simulink model "pll_hogge_lock"  (Simulink 6.6)
settings: Solver=ode23tb  StartTime=0.0  StopTime=200.0e-9  MaxStep=1.0e-12  RelTol=1e-4
values from neighbouring files (symbols this model uses):
  C1 = 2.2e-9    (= 2.2e-09)    [plot_bode_open_and_closed_2.m]    (also in plot_bode_open_and_closed_hogge.m)
  C2 = 1.0e-9    (= 1e-09)    [plot_bode_open_and_closed_1.m]    (also in plot_bode_open_and_closed_2.m = 3.3e-08; plot_bode_open_and_closed_hogge.m = 3.3e-08)
  R1 = 10000    [plot_bode_open_and_closed_1.m]
libraries: powerlib x8, simulink_extras x3, commsynccomp2 x1, simulink x1, dspswit3 x1
settings Model: Creator=Administrator  LastModifiedBy=Administrator

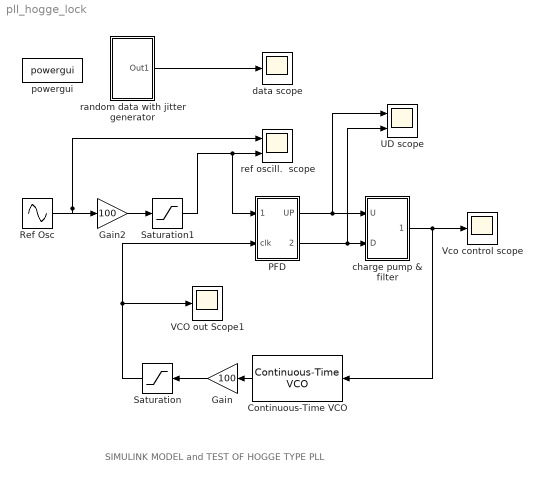
== system pll_hogge_lock ==
  note: SIMULINK MODEL and TEST OF HOGGE TYPE PLL
  " charge pump & filter" : Subsystem
  Continuous-Time VCO : commsynccomp2/Continuous-Time VCO  Orientation=left  SystemSampleTime=-1  Ac=1  Fc=1.999e9  Kc=500e6  Ph=-pi/2
  Gain : Gain  Orientation=left  Gain=100  RndMeth=Nearest
  Gain2 : Gain  Gain=100  RndMeth=Nearest
  PFD : Subsystem
  Ref Osc : Sin  Frequency=2*pi*1e9  Phase=3*pi/2  SampleTime=0
      settings: AttributesFormatString=%<Frequency> (rad/s)
  Saturation : Saturate  Orientation=left  UpperLimit=1  LowerLimit=0
  Saturation1 : Saturate  UpperLimit=1  LowerLimit=0
  UD scope : Scope  NumInputPorts=2
      settings: TimeRange=4.693877551020409e-008  YMin=-0.5~-0.5  YMax=1.5~1.5  SaveName=ScopeData5
  VCO out Scope1 : Scope
      settings: TimeRange=6.548881036513545e-009  YMin=-0.5  YMax=1.5  SaveName=ScopeData2  SampleTime=1e-8
  Vco control scope : Scope
      settings: TimeRange=2.564935064935065e-008  YMin=-0.8  YMax=1.2
  data scope : Scope
      settings: YMin=-0.5  YMax=1.5
  powergui : powerlib/powergui  SystemSampleTime=-1  SimulationMode=Continuous  SampleTime=50e-6  echomessages=off  RestoreLinks=warning  x0status=blocks  Frange=[0:2:500]  Ylog=off  Xlog=on  ShowGrid=off  save=off  variable=ZData  ZoomFFT=on  StartTime=0.0  cycles=1  DisplayStyle=1  fundamental=60  FreqAxis=off  MaxFrequency=1000  frequencyindice=0  frequencyindicesteady=1  RmsSteady=1  display=off  Ts=0  frequency=60  methode=off  HookPort=off  Interpol=off
  random data with jitter generator : Subsystem
  ref oscill.  scope : Scope  NumInputPorts=2
      settings: TimeRange=1.752837326607819e-008  YMin=-1.5~-0.5  YMax=1.5~1.5  SaveName=ScopeData3
  wires:
  random data with jitter generator/1(Out1) -> data scope/1
  Continuous-Time VCO/1 -> Gain/1
  PFD/1(UP) -> " charge pump & filter"/1(U), UD scope/1
  PFD/2(DN) -> " charge pump & filter"/2(D), UD scope/2
  " charge pump & filter"/1(contrl) -> Vco control scope/1, Continuous-Time VCO/1
  Ref Osc/1 -> ref oscill.  scope/1, Gain2/1
  Saturation/1 -> VCO out Scope1/1, PFD/2(clk)
  Gain/1 -> Saturation/1
  Saturation1/1 -> ref oscill.  scope/2, PFD/1(data)
  Gain2/1 -> Saturation1/1

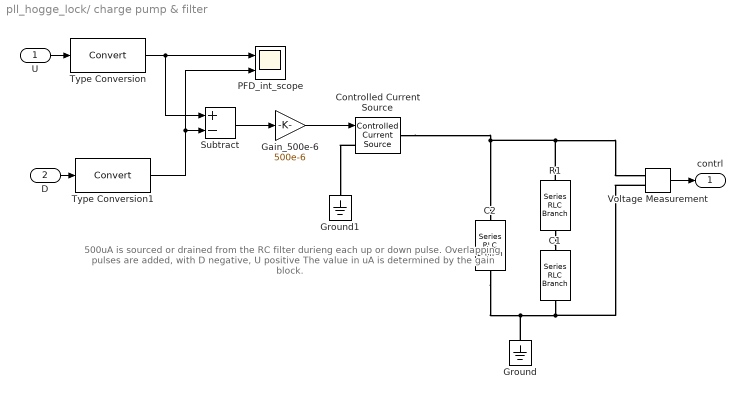
== system pll_hogge_lock/ charge pump & filter ==
  note: 500uA is sourced or drained from
      | the RC filter durieng each up or down
      | pulse. Overlapping pulses are added,
      | with D negative, U positive
      | The value in uA is determined by the gain block.
  U : Inport
  D : Inport  Port=2
  C1 : powerlib/Elements/Series RLC Branch  Orientation=down  DialogController=POWERSYS.PowerSysDialog  PhysicalDomain=powersysdomain  SubClassName=unknown  LeftPortType=p1  RightPortType=p1  LConnTagsString=__new0  RConnTagsString=__new0  BranchType=C  Resistance=1  Inductance=1e-3  SetiL0=off  InitialCurrent=0  Capacitance=C1  Setx0=on  InitialVoltage=0  Measurements=None
  C2 : powerlib/Elements/Series RLC Branch  Orientation=down  DialogController=POWERSYS.PowerSysDialog  PhysicalDomain=powersysdomain  SubClassName=unknown  LeftPortType=p1  RightPortType=p1  LConnTagsString=__new0  RConnTagsString=__new0  BranchType=C  Resistance=1  Inductance=1e-3  SetiL0=off  InitialCurrent=0  Capacitance=C2  Setx0=on  InitialVoltage=0  Measurements=None
  Controlled Current Source : powerlib/Electrical Sources/Controlled Current Source  DialogController=POWERSYS.PowerSysDialog  SystemSampleTime=-1  Initialize=on  Source_Type=DC  Amplitude=0  Phase=0  Frequency=0  Measurements=Current
  Gain_500e-6 : Gain  Gain=500e-6  RndMeth=Nearest
  Ground : powerlib/Elements/Ground  Orientation=down  DialogController=POWERSYS.PowerSysDialog  PhysicalDomain=powersysdomain  SubClassName=unknown  LeftPortType=p1  RightPortType=p1  LConnTagsString=a
  Ground1 : powerlib/Elements/Ground  Orientation=down  DialogController=POWERSYS.PowerSysDialog  PhysicalDomain=powersysdomain  SubClassName=unknown  LeftPortType=p1  RightPortType=p1  LConnTagsString=a
  PFD_int_scope : Scope  NumInputPorts=2
      settings: TimeRange=1e-007  YMin=-0.5~-0.5  YMax=1.5~1.5  SaveName=ScopeData7
  R1 : powerlib/Elements/Series RLC Branch  Orientation=down  DialogController=POWERSYS.PowerSysDialog  PhysicalDomain=powersysdomain  SubClassName=unknown  LeftPortType=p1  RightPortType=p1  LConnTagsString=__new0  RConnTagsString=__new0  BranchType=R  Resistance=R1  Inductance=1e-3  SetiL0=off  InitialCurrent=0  Capacitance=C1  Setx0=off  InitialVoltage=0  Measurements=None
  Subtract : Sum  Inputs=+-  OutDataTypeMode=double  OutScaling=2^-10  RndMeth=Nearest  InputSameDT=on
  Type Conversion : DataTypeConversion  OutDataTypeMode=double  RndMeth=Nearest
  Type Conversion1 : DataTypeConversion  OutDataTypeMode=double  RndMeth=Nearest
  Voltage Measurement : powerlib/Measurements/Voltage Measurement  DialogController=POWERSYS.PowerSysDialog  SystemSampleTime=-1  PhasorSimulation=off  OutputType=Complex  PSBequivalent=0
  contrl : Outport
  wires:
  Voltage Measurement/1 -> contrl/1
  Type Conversion1/1 -> Subtract/2, PFD_int_scope/2
  Type Conversion/1 -> Subtract/1, PFD_int_scope/1
  Gain_500e-6/1 -> Controlled Current Source/1
  Subtract/1 -> Gain_500e-6/1
  U/1 -> Type Conversion/1
  D/1 -> Type Conversion1/1
  connections:
  R1/RConn1 -- C1/LConn1
  Ground/LConn1 -- C1/RConn1 -- Voltage Measurement/LConn2 -- C2/RConn1
  R1/LConn1 -- Voltage Measurement/LConn1 -- C2/LConn1 -- Controlled Current Source/RConn1
  Controlled Current Source/LConn1 -- Ground1/LConn1

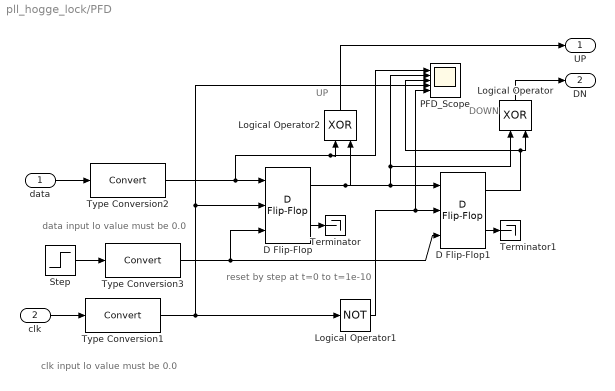
== system pll_hogge_lock/PFD ==
  note: DOWN
  note: UP
  note: clk input lo value must be 0.0
  note: data input lo value must be 0.0
  note: reset by step at t=0 to t=1e-10
  data : Inport
  clk : Inport  Port=2
  D Flip-Flop : simulink_extras/Flip Flops/D Flip-Flop  SystemSampleTime=-1
  D Flip-Flop1 : simulink_extras/Flip Flops/D Flip-Flop  SystemSampleTime=-1
  Logical Operator : Logic  Orientation=up  Operator=XOR  IconShape=distinctive
  Logical Operator1 : Logic  Operator=NOT  IconShape=distinctive
  Logical Operator2 : Logic  Orientation=up  Operator=XOR  IconShape=distinctive
  PFD_Scope : Scope  NumInputPorts=5
      settings: TimeRange=2.582029743641334e-009  YMin=-0.5~-0.5~-0.5~-0.5~-0.5  YMax=1.5~1.5~1.5~1.5~1.5  SaveName=ScopeData6
  Step : Step  Time=1.0e-10  Before=0.0  After=1.0  SampleTime=0  VectorParams1D=off  ZeroCross=off
  Terminator : Terminator
  Terminator1 : Terminator
  Type Conversion1 : DataTypeConversion  OutDataTypeMode=boolean  RndMeth=Nearest
  Type Conversion2 : DataTypeConversion  OutDataTypeMode=boolean  RndMeth=Nearest
  Type Conversion3 : DataTypeConversion  OutDataTypeMode=boolean  RndMeth=Nearest
  UP : Outport
  DN : Outport  Port=2
  wires:
  D Flip-Flop/2 -> Terminator/1
  D Flip-Flop1/2 -> Terminator1/1
  Logical Operator1/1 -> D Flip-Flop1/2, PFD_Scope/5
  D Flip-Flop/1 -> D Flip-Flop1/1, Logical Operator/1, PFD_Scope/2, Logical Operator2/2
  Type Conversion3/1 -> D Flip-Flop1/3, D Flip-Flop/3
  D Flip-Flop1/1 -> Logical Operator/2, PFD_Scope/3
  Type Conversion1/1 -> D Flip-Flop/2, PFD_Scope/4, Logical Operator1/1
  data/1 -> Type Conversion2/1
  clk/1 -> Type Conversion1/1
  Logical Operator2/1 -> UP/1
  Logical Operator/1 -> DN/1
  Type Conversion2/1 -> D Flip-Flop/1, Logical Operator2/1, PFD_Scope/1
  Step/1 -> Type Conversion3/1

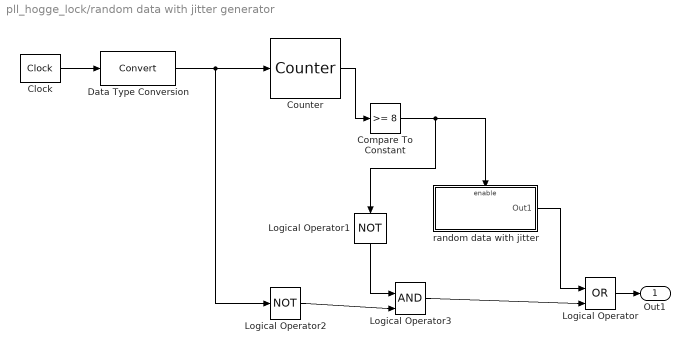
== system pll_hogge_lock/random data with jitter generator ==
  Clock : simulink_extras/Flip Flops/Clock  SystemSampleTime=-1  MaskParam1=1.0e-9
  Compare To Constant : simulink/Logic and Bit Operations/Compare To Constant  SystemSampleTime=-1  relop=>=  const=8  LogicOutDataTypeMode=uint8  ZeroCross=off
  Counter : dspswit3/Counter  Direction=Up  CountEvent=Rising edge  CounterSize=User defined  MaxCount=255  InitialCount=0  Output=Count  HitValue=8  ResetInput=off  SamplesPerFrame=1  Ts=1  CntDtype=double  HitDtype=Logical
  Data Type Conversion : DataTypeConversion  OutDataTypeMode=boolean  RndMeth=Nearest
  Logical Operator : Logic  Operator=OR  IconShape=distinctive  AllPortsSameDT=off  OutDataTypeMode=Boolean
  Logical Operator1 : Logic  Orientation=down  Operator=NOT  IconShape=distinctive  AllPortsSameDT=off  OutDataTypeMode=Boolean
  Logical Operator2 : Logic  Operator=NOT  IconShape=distinctive  AllPortsSameDT=off  OutDataTypeMode=Boolean
  Logical Operator3 : Logic  IconShape=distinctive  AllPortsSameDT=off  OutDataTypeMode=Boolean
  random data with jitter : Subsystem  TreatAsAtomicUnit=on
  Out1 : Outport
  wires:
  Counter/1 -> Compare To Constant/1
  Clock/1 -> Data Type Conversion/1
  Compare To Constant/1 -> Logical Operator1/1, random data with jitter/Enable
  Data Type Conversion/1 -> Counter/1, Logical Operator2/1
  Logical Operator3/1 -> Logical Operator/2
  random data with jitter/1(Out1) -> Logical Operator/1
  Logical Operator2/1 -> Logical Operator3/2
  Logical Operator1/1 -> Logical Operator3/1
  Logical Operator/1 -> Out1/1

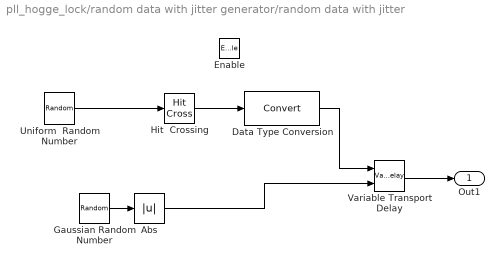
== system pll_hogge_lock/random data with jitter generator/random data with jitter ==
  Enable : EnablePort
  Abs : Abs
  Data Type Conversion : DataTypeConversion  OutDataTypeMode=double  RndMeth=Nearest
  Gaussian Random Number : RandomNumber  Variance=6.25e-20  Seed=2316  SampleTime=[1e-9 0]
  Hit  Crossing : HitCross  HitCrossingOffset=0.5  SampleTime=[1.0e-9 0]
  Uniform  Random Number : UniformRandomNumber  Minimum=0  Seed=314159265  SampleTime=[1.0e-9 0]
  Variable Transport Delay : VariableTransportDelay  MaximumDelay=0.8e-9  MaximumPoints=8192  ZeroDelay=on
  Out1 : Outport
  wires:
  Uniform  Random Number/1 -> Hit  Crossing/1
  Gaussian Random Number/1 -> Abs/1
  Hit  Crossing/1 -> Data Type Conversion/1
  Data Type Conversion/1 -> Variable Transport Delay/1
  Abs/1 -> Variable Transport Delay/2
  Variable Transport Delay/1 -> Out1/1
